simulink model "teste_linearizado_apos_swing"  (R2017b)
settings: Solver=VariableStepAuto  StartTime=0.0  StopTime=1  MaxStep=0.001  RelTol=1e-3
undefined symbols (not defined in the file or in its folder): entradas3
settings Model: Creator=Enrique Pinto  LastModifiedBy=Enrique Pinto

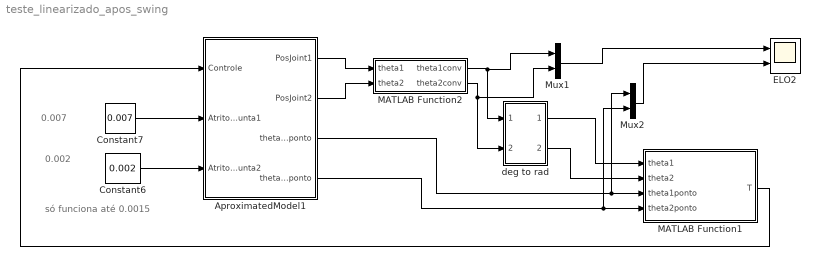
== system teste_linearizado_apos_swing ==
  note: só funciona até 0.0015
  note: 0.007
  note: 0.002
  AproximatedModel1 : Subsystem
  Constant6 : Constant  Value=0.002
  Constant7 : Constant  Value=0.007
  ELO2 : Scope  NumInputPorts=2
  MATLAB Function1 : MATLAB Function  TreatAsAtomicUnit=on
  MATLAB Function2 : MATLAB Function  TreatAsAtomicUnit=on
  Mux1 : Mux  Inputs=2
  Mux2 : Mux  Inputs=2
  deg to rad : Subsystem
  wires:
  Mux2/1 -> ELO2/2
  AproximatedModel1/1(PosJoint1) -> MATLAB Function2/1(theta1)
  MATLAB Function2/1(theta1conv) -> Mux1/1, deg to rad/1(In1)
  AproximatedModel1/2(PosJoint2) -> MATLAB Function2/2(theta2)
  deg to rad/1(Out1) -> MATLAB Function1/1(theta1)
  MATLAB Function1/1(T) -> AproximatedModel1/1(Controle)
  deg to rad/2(Out2) -> MATLAB Function1/2(theta2)
  MATLAB Function2/2(theta2conv) -> Mux1/2, deg to rad/2(In2)
  AproximatedModel1/4(theta2ponto) -> MATLAB Function1/4(theta2ponto), Mux2/2
  Constant6/1 -> AproximatedModel1/3(AtritoJunta2)
  AproximatedModel1/3(theta1ponto) -> Mux2/1, MATLAB Function1/3(theta1ponto)
  Constant7/1 -> AproximatedModel1/2(AtritoJunta1)
  Mux1/1 -> ELO2/1

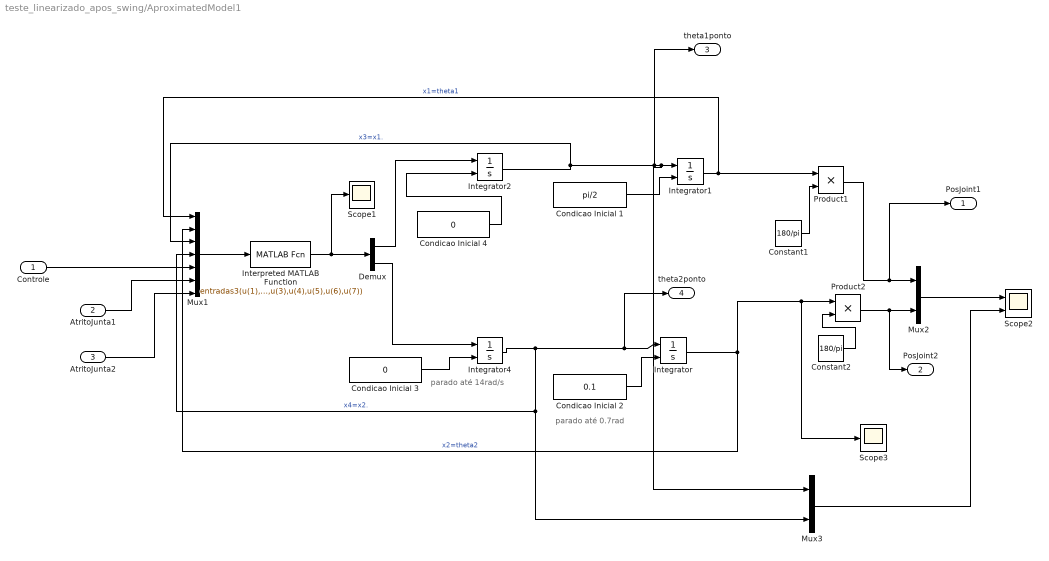
== system teste_linearizado_apos_swing/AproximatedModel1 ==
  note: parado até 14rad/s
  note: parado até 0.7rad
  Controle : Inport
  AtritoJunta1 : Inport  Port=2
  AtritoJunta2 : Inport  Port=3
  Condicao Inicial 1 : Constant  Value=pi/2
  Condicao Inicial 2 : Constant  Value=0.1
  Condicao Inicial 3 : Constant  Value=0
  Condicao Inicial 4 : Constant  Value=0
  Constant1 : Constant  Value=180/pi
  Constant2 : Constant  Value=180/pi
  Demux : Demux  Outputs=2
  Integrator : Integrator  InitialConditionSource=external  InitialCondition=pi+1
  Integrator1 : Integrator  InitialConditionSource=external
  Integrator2 : Integrator  InitialConditionSource=external  InitialCondition=-6
  Integrator4 : Integrator  InitialConditionSource=external  InitialCondition=12
  Interpreted MATLAB Function : MATLABFcn  MATLABFcn=entradas3(u(1),u(2),u(3),u(4),u(5),u(6),u(7))  OutputDimensions=2  OutputSignalType=real
  Mux1 : Mux  Inputs=7
  Mux2 : Mux  Inputs=2
  Mux3 : Mux  Inputs=2
  Product1 : Product
  Product2 : Product
  Scope1 : Scope
  Scope2 : Scope  NumInputPorts=2
  Scope3 : Scope
  PosJoint1 : Outport
  PosJoint2 : Outport  Port=2
  theta1ponto : Outport  Port=3
  theta2ponto : Outport  Port=4
  wires:
  AtritoJunta2/1 -> Mux1/7
  AtritoJunta1/1 -> Mux1/6
  Mux1/1 -> Interpreted MATLAB Function/1
  Demux/2 -> Integrator4/1
  Demux/1 -> Integrator2/1
  Integrator1/1 -> Product1/1, Mux1/1  "x1=theta1"
  Integrator4/1 -> theta2ponto/1, Integrator/1, Mux3/2, Mux1/4  "x4=x2."
  Integrator/1 -> Scope3/1, Product2/1, Mux1/2  "x2=theta2"
  Condicao Inicial 2/1 -> Integrator/2
  Integrator2/1 -> theta1ponto/1, Mux3/1, Integrator1/1, Mux1/3  "x3=x1."
  Mux2/1 -> Scope2/1
  Condicao Inicial 1/1 -> Integrator1/2
  Controle/1 -> Mux1/5
  Constant1/1 -> Product1/2
  Product1/1 -> PosJoint1/1, Mux2/1
  Constant2/1 -> Product2/2
  Product2/1 -> PosJoint2/1, Mux2/2
  Interpreted MATLAB Function/1 -> Scope1/1, Demux/1
  Condicao Inicial 3/1 -> Integrator4/2
  Condicao Inicial 4/1 -> Integrator2/2
  Mux3/1 -> Scope2/2

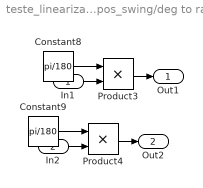
== system teste_linearizado_apos_swing/deg to rad ==
  In1 : Inport
  In2 : Inport  Port=2
  Constant8 : Constant  Value=pi/180
  Constant9 : Constant  Value=pi/180
  Product3 : Product
  Product4 : Product
  Out1 : Outport
  Out2 : Outport  Port=2
  wires:
  Constant9/1 -> Product4/1
  Constant8/1 -> Product3/1
  In1/1 -> Product3/2
  In2/1 -> Product4/2
  Product4/1 -> Out2/1
  Product3/1 -> Out1/1

== matlab function teste_linearizado_apos_swing/MATLAB Function1 ==
  data: theta1 input; T output; theta2 input; theta1ponto input; theta2ponto input
function T = controle_lin(theta1,theta2,theta1ponto,theta2ponto)
g=9.81;
m1=0.0555; 
m2=0.0416; 
L1=0.168;
l1=0.0973; 
L2=0.140;
l2=0.07;
I1=1.97e-4;
I2=9.58e-5;
 
%% Matriz de Inércia

 m11=I1+I2+m1*l1^2+m2*(L1^2+l2^2+2*L1*l2*cos(theta2));
 m12=I2+m2*(l2^2+L1*l2*cos(theta2));
 m21=m12;
 m22=I2+m2*l2^2;

 %% Matriz correspondente as forças exercidas pela gravidade

G = [(m1*l1+m2*L1)*g*cos(theta1)+m2*l2*g*cos(theta1+theta2);
     m2*l2*g*cos(theta1+theta2)];

%% Matriz correspondente as forças de Coriolis e centrifuga

h=m2*L1*l2*sin(theta2);

H = [-h*(2*theta1ponto*theta2ponto+(theta2ponto^2))+G(1);
    h*(theta1ponto^2)+G(2)];
%% Controle

%Realimentação Linearizante
% kp=150;
% kd=13;
% 
% u=kp*(pi/2-theta1)-kd*theta1ponto;
% alpha=(m12*H(2)/m22)-H(1);
% beta=(m11-((m12^2)/m22));
% T=double([(beta*u-alpha)]);

% Controle Linearizado
x=[theta1;theta2;theta1ponto;theta2ponto];
xlin=[pi/2;0;0;0];
K=[25.038844779283560 29.002032918917394 4.329388916638663 0.881420311713631];
T=-K*(x-xlin);

== matlab function teste_linearizado_apos_swing/MATLAB Function2 ==
  data: theta1 input; theta1conv output; theta2 input; theta2conv output
function [theta1conv,theta2conv] = angle_convert(theta1,theta2)
theta1_360=mod(theta1,360);
if theta1_360>180
    theta1conv=theta1_360-360;  
else
    theta1conv=theta1_360;
end
theta2_360=mod(theta2,360);
if theta2_360>180
    theta2conv=theta2_360-360;  
else
    theta2conv=theta2_360;
end
